simulink model "Skogestad"  (R2023b)
settings: Solver=VariableStepAuto  StartTime=0.0  StopTime=5  RelTol=1e-8
values from neighbouring files (symbols this model uses):
  D_hiv_fart = [M(3),rho_vann*Cd*A_z*Z_2]    [Alternative_Parameter.m]
settings Model: Creator=Anne Brit  LastModifiedBy=anneb

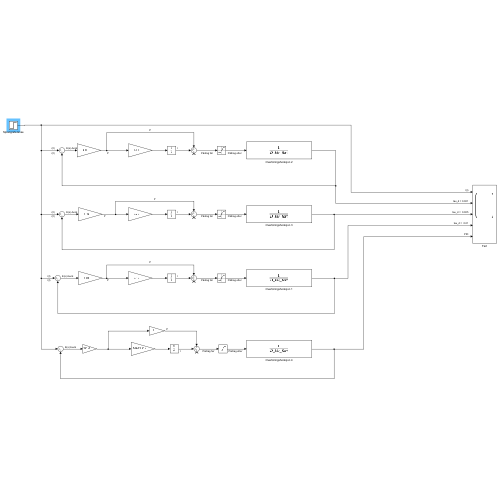
[thumbnail: Simulink's stored preview of the top-level diagram]
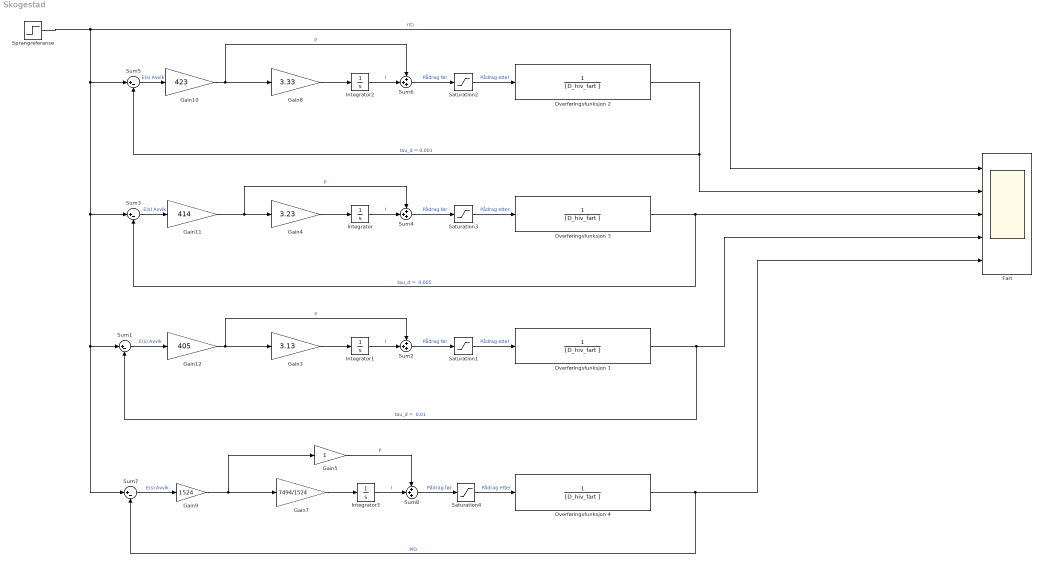
== system Skogestad ==
  Fart : Scope  NumInputPorts=5
  Gain10 : Gain  Gain=423
  Gain11 : Gain  Gain=414
  Gain12 : Gain  Gain=405
  Gain3 : Gain  Gain=3.13
  Gain4 : Gain  Gain=3.23
  Gain5 : Gain
  Gain7 : Gain  Gain=7494/1524
  Gain8 : Gain  Gain=3.33
  Gain9 : Gain  Gain=1524
  Integrator{,1..3} (4 alike) : Integrator
  Overføringsfunksjon {1..4} (4 alike) : TransferFcn  Denominator=[D_hiv_fart ]
  Saturation{1..4} (4 alike) : Saturate  UpperLimit=115  LowerLimit=-145
  Sprangreferanse : Step  After=0.0325  SampleTime=0
  Sum{1,3,5,7} (4 alike) : Sum  Inputs=|+-
  Sum{2,4,6,8} (4 alike) : Sum  Inputs=+++
  wires:
  Sum3/1 -> Gain11/1  "E(s) Avvik"
  Integrator/1 -> Sum4/2  "I"
  Overføringsfunksjon 3/1 -> Sum3/2, Fart/3  "tau_d =  0.005"
  Sum4/1 -> Saturation3/1  "Pådrag før"
  Saturation3/1 -> Overføringsfunksjon 3/1  "Pådrag etter"
  Gain4/1 -> Integrator/1
  Gain3/1 -> Integrator1/1
  Saturation1/1 -> Overføringsfunksjon 1/1  "Pådrag etter"
  Sum2/1 -> Saturation1/1  "Pådrag før"
  Overføringsfunksjon 1/1 -> Fart/4, Sum1/2  "tau_d =  0.01"
  Sum1/1 -> Gain12/1  "E(s) Avvik"
  Integrator1/1 -> Sum2/2  "I"
  Gain8/1 -> Integrator2/1
  Saturation2/1 -> Overføringsfunksjon 2/1  "Pådrag etter"
  Sum6/1 -> Saturation2/1  "Pådrag før"
  Overføringsfunksjon 2/1 -> Sum5/2, Fart/2  "tau_d = 0.001"
  Sum5/1 -> Gain10/1  "E(s) Avvik"
  Integrator2/1 -> Sum6/2  "I"
  Gain5/1 -> Sum8/1  "P"
  Sum7/1 -> Gain9/1  "E(s) Avvik"
  Gain9/1 -> Gain5/1, Gain7/1
  Gain7/1 -> Integrator3/1
  Integrator3/1 -> Sum8/2  "I"
  Sum8/1 -> Saturation4/1  "Pådrag før"
  Saturation4/1 -> Overføringsfunksjon 4/1  "Pådrag etter"
  Overføringsfunksjon 4/1 -> Sum7/2, Fart/5  "PID"
  Gain10/1 -> Sum6/1, Gain8/1  "P"
  Gain11/1 -> Sum4/1, Gain4/1  "P"
  Gain12/1 -> Sum2/1, Gain3/1  "P"
  Sprangreferanse/1 -> Sum7/1, Sum1/1, Sum3/1, Sum5/1, Fart/1  "r(t)"
